simulink model "seat_heating_control"  (R2023b)
settings: Solver=FixedStepDiscrete  StartTime=0.0  StopTime=10.0  FixedStep=0.01  RelTol=1e-3
values from neighbouring files (symbols this model uses):
  RTE_OK = Simulink.Parameter    [init.m]
  TemperatureRanges_High = AUTOSAR.Parameter    [init.m]
  TemperatureRanges_Low = AUTOSAR.Parameter    [init.m]
  TemperatureRanges_Medium = AUTOSAR.Parameter    [init.m]
undefined symbols (not defined in the file or in its folder): HeatingActivate_SetHeatingCoil, IDT_PowerState, temp
settings Model: Creator=nabilekhoury  LastModifiedBy=developer
settings SolverCC: AlgebraicLoopSolver=TrustRegion
settings DataIOCC: SaveFormat=StructureWithTime
settings OptimizationCC: DefaultParameterBehavior=Inlined  EnhancedBackFolding=on  PassReuseOutputArgsAs=Individual arguments  ZeroExternalMemoryAtStartup=off  ZeroInternalMemoryAtStartup=off  OptimizeBlockOrder=speed  DifferentSizesBufferReuse=on  OptimizationCustomize=off  EfficientTunableParamExpr=on
settings DebuggingCC: ParameterTunabilityLossMsg=error  UnconnectedInputMsg=warning  UnconnectedOutputMsg=warning  UnconnectedLineMsg=warning  ArithmeticOperatorsInVariantConditions=warning
settings ModelReferenceCC: EnableRefExpFcnMdlSchedulingChecks=on  ModelReferenceNumInstancesAllowed=Single
settings SFSimCC: MATLABDynamicMemAlloc=off  CustomCodeUndefinedFunction=UseInterfaceOnly
settings RTWCC: Description=AUTOSAR  SystemTargetFile=autosar.tlc  GenCodeOnly=on  TemplateMakefile=ert_default_tmf  GenerateReport=on  IncludeHyperlinkInReport=on  LaunchReport=on  DataTypeReplacement=CDataTypesFixedWidth  GenerateTraceInfo=on  GenerateTraceReport=on  GenerateTraceReportSl=on  GenerateTraceReportSf=on  GenerateTraceReportEml=on
settings CodeAppCC: ForceParamTrailComments=on  IgnoreCustomStorageClasses=off  OperatorAnnotations=on  SimulinkDataObjDesc=on  SFDataObjDesc=on  InsertBlockDesc=on
settings STFCustomTargetCC: MultiwordLength=256  ParMdlRefBuildCompliant=on  CompOptLevelCompliant=on  IncludeMdlTerminateFcn=off  CombineOutputUpdateFcns=on  SuppressErrorStatus=on  ERTCustomFileBanners=on  SupportNonFinite=off  SupportComplex=off  SupportContinuousTime=off  SupportNonInlinedSFcns=off  RemoveResetFunc=on  MATLABClassNameForMDSCustomization=Simulink.SoftwareTarget.ERTCustomization  AutosarCompliant=on  UseToolchainInfoCompliant=on  LookupTableObjectStructAxisOrder=2,1,3,4,...  LUTObjectStructOrderEvenSpacing=Size,Table,Breakpoints  SystemTargetFile=autosar.tlc
settings ERTTargetCC: TargetLangStandard=C99 (ISO)  ConcurrentExecutionCompliant=off  IncludeMdlTerminateFcn=off  SuppressErrorStatus=on  SupportNonFinite=off  SupportComplex=off  ModelStepFunctionPrototypeControlCompliant=off  CPPClassGenCompliant=off  AutosarCompliant=on  LookupTableObjectStructAxisOrder=2,1,3,4,...  LUTObjectStructOrderEvenSpacing=Size,Table,Breakpoints  InlinedParameterPlacement=NonHierarchical  ERTCustomFileTemplate=example_file_process.tlc  BooleanTrueId=TRUE  BooleanFalseId=FALSE

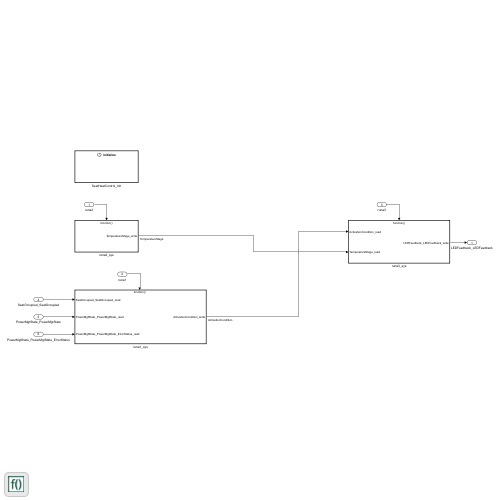
[thumbnail: Simulink's stored preview of the top-level diagram]
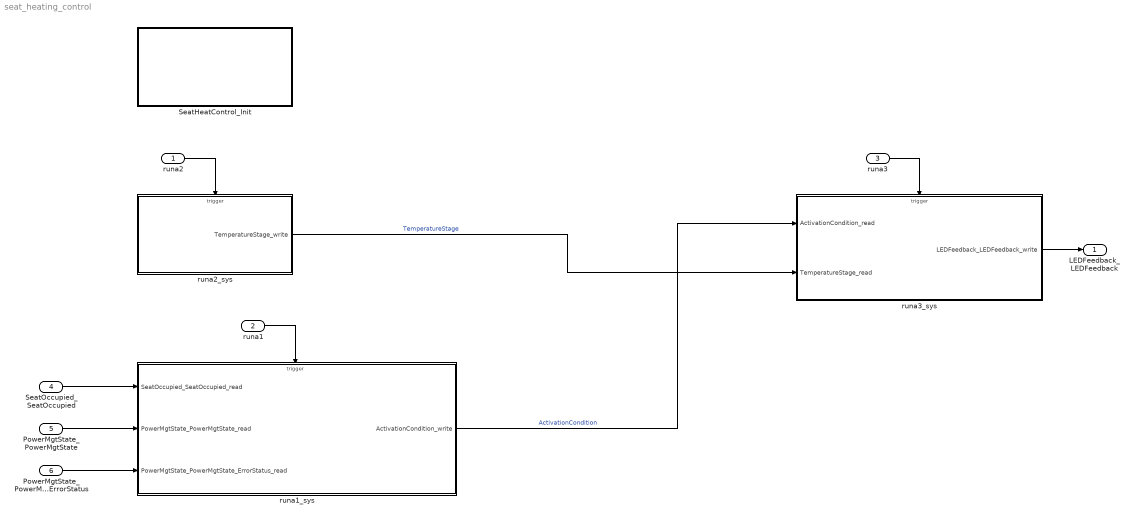
== system seat_heating_control ==
  runa2 : Inport  SampleTime=0.01  OutputFunctionCall=on
  runa1 : Inport  Port=2  SampleTime=0.01  OutputFunctionCall=on
  runa3 : Inport  Port=3  SampleTime=0.01  OutputFunctionCall=on
  SeatOccupied_SeatOccupied : Inport  Port=4  OutDataTypeStr=IDT_SeatStatus  PortDimensions=1
  PowerMgtState_PowerMgtState : Inport  Port=5  OutDataTypeStr=Enum: IDT_PowerState  PortDimensions=1
  PowerMgtState_PowerMgtState_ErrorStatus : Inport  Port=6  OutDataTypeStr=uint8  PortDimensions=1
  SeatHeatControl_Init : Subsystem
  runa1_sys : Subsystem
  runa2_sys : Subsystem
  runa3_sys : Subsystem
  LEDFeedback_LEDFeedback : Outport  OutDataTypeStr=boolean  PortDimensions=3
  wires:
  SeatOccupied_SeatOccupied/1 -> runa1_sys/1(SeatOccupied_SeatOccupied_read)
  PowerMgtState_PowerMgtState/1 -> runa1_sys/2(PowerMgtState_PowerMgtState_read)
  PowerMgtState_PowerMgtState_ErrorStatus/1 -> runa1_sys/3(PowerMgtState_PowerMgtState_ErrorStatus_read)
  runa3_sys/1(LEDFeedback_LEDFeedback_write) -> LEDFeedback_LEDFeedback/1
  runa2_sys/1(TemperatureStage_write) -> runa3_sys/2(TemperatureStage_read)  "TemperatureStage"
  runa1_sys/1(ActivationCondition_write) -> runa3_sys/1(ActivationCondition_read)  "ActivationCondition"
  runa2/1 -> runa2_sys/Trigger
  runa1/1 -> runa1_sys/Trigger
  runa3/1 -> runa3_sys/Trigger

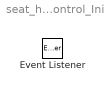
== system seat_heating_control/SeatHeatControl_Init ==
  Event Listener : EventListener  EventName=reset

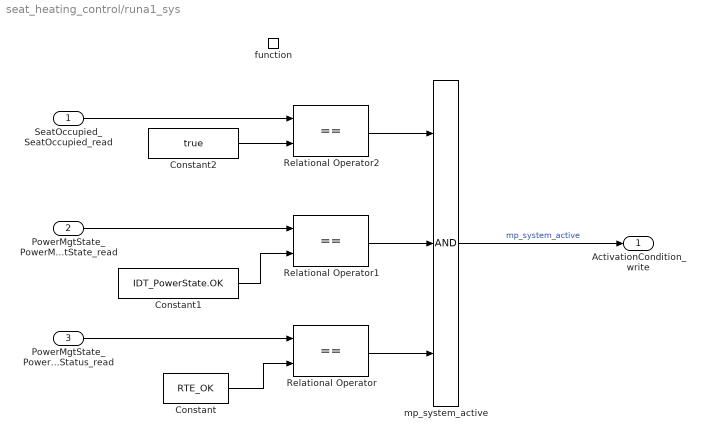
== system seat_heating_control/runa1_sys ==
  SeatOccupied_SeatOccupied_read : Inport
  PowerMgtState_PowerMgtState_read : Inport  Port=2
  PowerMgtState_PowerMgtState_ErrorStatus_read : Inport  Port=3
  function : TriggerPort  TriggerType=function-call  VariantControl=(inherit)  SampleTimeType=periodic  SampleTime=-1
  Constant : Constant  Value=RTE_OK
  Constant1 : Constant  Value=IDT_PowerState.OK
  Constant2 : Constant  Value=true
  Relational Operator : RelationalOperator  Operator===  OutDataTypeStr=boolean  RndMeth=Simplest  InputSameDT=off
  Relational Operator1 : RelationalOperator  Operator===  OutDataTypeStr=boolean  RndMeth=Simplest  InputSameDT=off
  Relational Operator2 : RelationalOperator  Operator===  OutDataTypeStr=boolean  RndMeth=Simplest  InputSameDT=off
  mp_system_active : Logic  Inputs=3  AllPortsSameDT=off  OutDataTypeStr=boolean
  ActivationCondition_write : Outport  OutDataTypeStr=boolean  PortDimensions=1  InitialOutput=0
  wires:
  mp_system_active/1 -> ActivationCondition_write/1  "mp_system_active"
  PowerMgtState_PowerMgtState_ErrorStatus_read/1 -> Relational Operator/1
  PowerMgtState_PowerMgtState_read/1 -> Relational Operator1/1
  Constant2/1 -> Relational Operator2/2
  SeatOccupied_SeatOccupied_read/1 -> Relational Operator2/1
  Relational Operator2/1 -> mp_system_active/1
  Constant1/1 -> Relational Operator1/2
  Relational Operator/1 -> mp_system_active/3
  Relational Operator1/1 -> mp_system_active/2
  Constant/1 -> Relational Operator/2

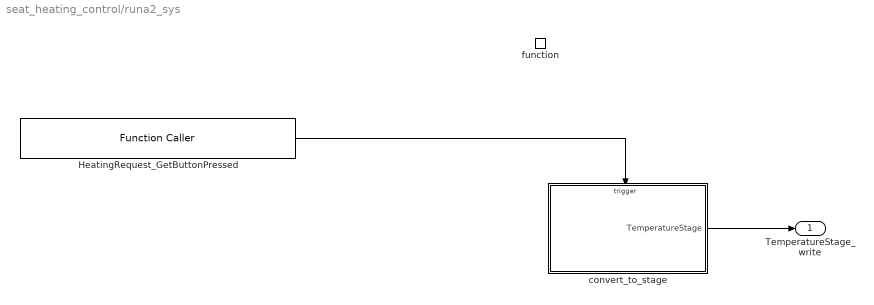
== system seat_heating_control/runa2_sys ==
  function : TriggerPort  TriggerType=function-call  VariantControl=(inherit)  SampleTimeType=periodic  SampleTime=-1
  HeatingRequest_GetButtonPressed : FunctionCaller  FunctionPrototype=status = HeatingRequest_GetButtonPressed()  OutputArgumentSpecifications=P_IDT_ButtonStatus
  convert_to_stage : Subsystem
  TemperatureStage_write : Outport  OutDataTypeStr=uint8  PortDimensions=1  InitialOutput=0
  wires:
  convert_to_stage/1(TemperatureStage) -> TemperatureStage_write/1
  HeatingRequest_GetButtonPressed/1 -> convert_to_stage/Trigger

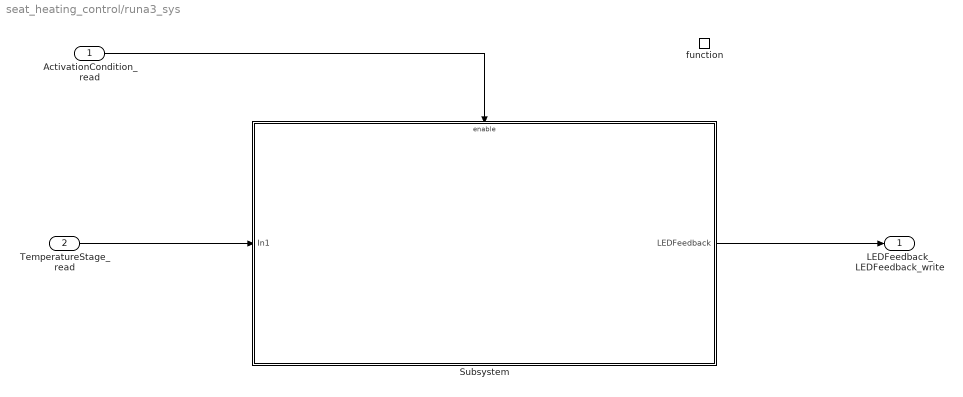
== system seat_heating_control/runa3_sys ==
  ActivationCondition_read : Inport
  TemperatureStage_read : Inport  Port=2
  function : TriggerPort  TriggerType=function-call  VariantControl=(inherit)  SampleTimeType=periodic  SampleTime=-1
  Subsystem : Subsystem
  LEDFeedback_LEDFeedback_write : Outport
      settings: EnsureOutportIsVirtual=on
  wires:
  ActivationCondition_read/1 -> Subsystem/Enable
  TemperatureStage_read/1 -> Subsystem/1(In1)
  Subsystem/1(LEDFeedback) -> LEDFeedback_LEDFeedback_write/1

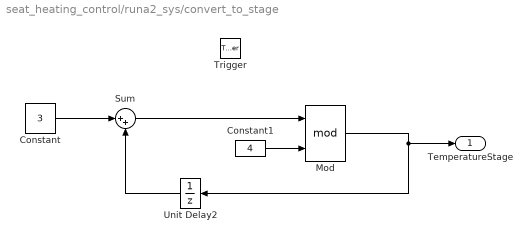
== system seat_heating_control/runa2_sys/convert_to_stage ==
  Trigger : TriggerPort  VariantControl=Variant  PortDimensions=1
  Constant : Constant  Value=3  OutDataTypeStr=Inherit: Inherit via back propagation
  Constant1 : Constant  Value=4  OutDataTypeStr=Inherit: Inherit via back propagation
  Mod : Math  Operator=mod
  Sum : Sum  Inputs=|++
  Unit Delay2 : UnitDelay  SampleTime=-1  HasFrameUpgradeWarning=on
      settings: AttributesFormatString=Init = %<InitialCondition>
  TemperatureStage : Outport  InitialOutput=0
  wires:
  Mod/1 -> TemperatureStage/1, Unit Delay2/1
  Unit Delay2/1 -> Sum/2
  Constant1/1 -> Mod/2
  Sum/1 -> Mod/1
  Constant/1 -> Sum/1

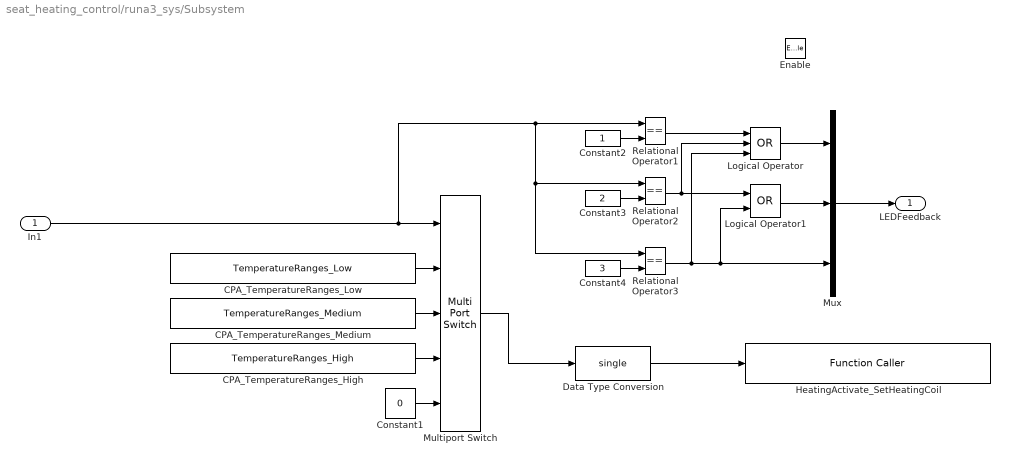
== system seat_heating_control/runa3_sys/Subsystem ==
  In1 : Inport
  Enable : EnablePort
  CPA_TemperatureRanges_High : Constant  Value=TemperatureRanges_High
  CPA_TemperatureRanges_Low : Constant  Value=TemperatureRanges_Low
  CPA_TemperatureRanges_Medium : Constant  Value=TemperatureRanges_Medium
  Constant1 : Constant  Value=0
  Constant2 : Constant  OutDataTypeStr=Inherit: Inherit via back propagation
  Constant3 : Constant  Value=2  OutDataTypeStr=Inherit: Inherit via back propagation
  Constant4 : Constant  Value=3  OutDataTypeStr=Inherit: Inherit via back propagation
  Data Type Conversion : DataTypeConversion  OutDataTypeStr=single  SaturateOnIntegerOverflow=off  RndMeth=Floor
  HeatingActivate_SetHeatingCoil : FunctionCaller  FunctionPrototype=HeatingActivate_SetHeatingCoil(temp)  InputArgumentSpecifications=single(1)
  Logical Operator : Logic  Operator=OR  Inputs=3  AllPortsSameDT=off  OutDataTypeStr=boolean
  Logical Operator1 : Logic  Operator=OR  AllPortsSameDT=off  OutDataTypeStr=boolean
  Multiport Switch : MultiPortSwitch  DataPortIndices={0,1,2,3}  DataPortForDefault=Additional data port  DiagnosticForDefault=None  OutDataTypeStr=IDT_Temperature  SaturateOnIntegerOverflow=off  InputSameDT=off
  Mux : Mux  Inputs=3
  Relational Operator1 : RelationalOperator  Operator===  OutDataTypeStr=boolean  RndMeth=Simplest  InputSameDT=off
  Relational Operator2 : RelationalOperator  Operator===  OutDataTypeStr=boolean  RndMeth=Simplest  InputSameDT=off
  Relational Operator3 : RelationalOperator  Operator===  OutDataTypeStr=boolean  RndMeth=Simplest  InputSameDT=off
  LEDFeedback : Outport
  wires:
  In1/1 -> Relational Operator3/1, Relational Operator2/1, Relational Operator1/1, Multiport Switch/1
  Constant2/1 -> Relational Operator1/2
  Constant4/1 -> Relational Operator3/2
  Mux/1 -> LEDFeedback/1
  CPA_TemperatureRanges_Medium/1 -> Multiport Switch/3
  Relational Operator2/1 -> Logical Operator1/1, Logical Operator/2
  Relational Operator1/1 -> Logical Operator/1
  Constant3/1 -> Relational Operator2/2
  Relational Operator3/1 -> Logical Operator/3, Logical Operator1/2, Mux/3
  Multiport Switch/1 -> Data Type Conversion/1
  Constant1/1 -> Multiport Switch/5
  CPA_TemperatureRanges_High/1 -> Multiport Switch/4
  CPA_TemperatureRanges_Low/1 -> Multiport Switch/2
  Logical Operator/1 -> Mux/1
  Logical Operator1/1 -> Mux/2
  Data Type Conversion/1 -> HeatingActivate_SetHeatingCoil/1
